simulink model "prova_ottimizzatore"  (R2018a)
settings: Solver=VariableStepAuto  StartTime=0.0  StopTime=10.0  RelTol=1e-3
settings Model: Creator=root  LastModifiedBy=root

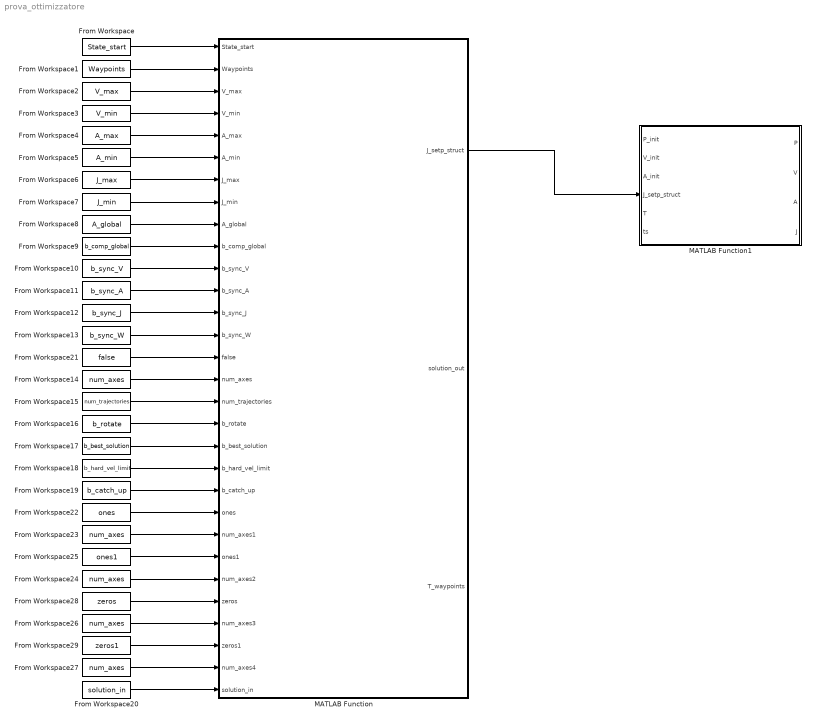
== system prova_ottimizzatore ==
  From Workspace : FromWorkspace  VariableName=State_start  SampleTime=0
  From Workspace1 : FromWorkspace  VariableName=Waypoints  SampleTime=0
  From Workspace10 : FromWorkspace  VariableName=b_sync_V  SampleTime=0
  From Workspace11 : FromWorkspace  VariableName=b_sync_A  SampleTime=0
  From Workspace12 : FromWorkspace  VariableName=b_sync_J  SampleTime=0
  From Workspace13 : FromWorkspace  VariableName=b_sync_W  SampleTime=0
  From Workspace{14,23..24,26..27} (5 alike) : FromWorkspace  VariableName=num_axes  SampleTime=0
  From Workspace15 : FromWorkspace  VariableName=num_trajectories  SampleTime=0
  From Workspace16 : FromWorkspace  VariableName=b_rotate  SampleTime=0
  From Workspace17 : FromWorkspace  VariableName=b_best_solution  SampleTime=0
  From Workspace18 : FromWorkspace  VariableName=b_hard_vel_limit  SampleTime=0
  From Workspace19 : FromWorkspace  VariableName=b_catch_up  SampleTime=0
  From Workspace2 : FromWorkspace  VariableName=V_max  SampleTime=0
  From Workspace20 : FromWorkspace  VariableName=solution_in  SampleTime=0
  From Workspace21 : FromWorkspace  VariableName=false  SampleTime=0
  From Workspace22 : FromWorkspace  VariableName=ones  SampleTime=0
  From Workspace25 : FromWorkspace  VariableName=ones1  SampleTime=0
  From Workspace28 : FromWorkspace  VariableName=zeros  SampleTime=0
  From Workspace29 : FromWorkspace  VariableName=zeros1  SampleTime=0
  From Workspace3 : FromWorkspace  VariableName=V_min  SampleTime=0
  From Workspace4 : FromWorkspace  VariableName=A_max  SampleTime=0
  From Workspace5 : FromWorkspace  VariableName=A_min  SampleTime=0
  From Workspace6 : FromWorkspace  VariableName=J_max  SampleTime=0
  From Workspace7 : FromWorkspace  VariableName=J_min  SampleTime=0
  From Workspace8 : FromWorkspace  VariableName=A_global  SampleTime=0
  From Workspace9 : FromWorkspace  VariableName=b_comp_global  SampleTime=0
  MATLAB Function : MATLAB Function  TreatAsAtomicUnit=on
  MATLAB Function1 : MATLAB Function  TreatAsAtomicUnit=on
  wires:
  From Workspace/1 -> MATLAB Function/1(State_start)
  From Workspace1/1 -> MATLAB Function/2(Waypoints)
  From Workspace2/1 -> MATLAB Function/3(V_max)
  From Workspace3/1 -> MATLAB Function/4(V_min)
  From Workspace4/1 -> MATLAB Function/5(A_max)
  From Workspace5/1 -> MATLAB Function/6(A_min)
  From Workspace6/1 -> MATLAB Function/7(J_max)
  From Workspace7/1 -> MATLAB Function/8(J_min)
  From Workspace8/1 -> MATLAB Function/9(A_global)
  From Workspace9/1 -> MATLAB Function/10(b_comp_global)
  From Workspace10/1 -> MATLAB Function/11(b_sync_V)
  From Workspace11/1 -> MATLAB Function/12(b_sync_A)
  From Workspace12/1 -> MATLAB Function/13(b_sync_J)
  From Workspace13/1 -> MATLAB Function/14(b_sync_W)
  From Workspace14/1 -> MATLAB Function/16(num_axes)
  From Workspace15/1 -> MATLAB Function/17(num_trajectories)
  From Workspace16/1 -> MATLAB Function/18(b_rotate)
  From Workspace17/1 -> MATLAB Function/19(b_best_solution)
  From Workspace18/1 -> MATLAB Function/20(b_hard_vel_limit)
  From Workspace19/1 -> MATLAB Function/21(b_catch_up)
  From Workspace20/1 -> MATLAB Function/30(solution_in)
  From Workspace21/1 -> MATLAB Function/15(false)
  From Workspace22/1 -> MATLAB Function/22(ones)
  From Workspace23/1 -> MATLAB Function/23(num_axes1)
  From Workspace24/1 -> MATLAB Function/25(num_axes2)
  From Workspace25/1 -> MATLAB Function/24(ones1)
  From Workspace26/1 -> MATLAB Function/27(num_axes3)
  From Workspace27/1 -> MATLAB Function/29(num_axes4)
  From Workspace28/1 -> MATLAB Function/26(zeros)
  From Workspace29/1 -> MATLAB Function/28(zeros1)
  MATLAB Function/1(J_setp_struct) -> MATLAB Function1/4(J_setp_struct)

== matlab function prova_ottimizzatore/MATLAB Function1 ==
  data: P_init input; P output; V_init input; A_init input; J_setp_struct input; T input; ts input; V output; A output; J output
function [P,V,A,J] = rollout(P_init,V_init,A_init,J_setp_struct,T,ts)

== matlab function prova_ottimizzatore/MATLAB Function ==
  data: State_start input; J_setp_struct output; Waypoints input; V_max input; V_min input; A_max input; A_min input; J_max input; J_min input; A_global input; b_comp_global input; b_sync_V input; b_sync_A input; b_sync_J input; b_sync_W input; false input; num_axes input; num_trajectories input; b_rotate input; b_best_solution input; b_hard_vel_limit input; b_catch_up input; ones input; num_axes1 input; ones1 input; num_axes2 input; zeros input; num_axes3 input; zeros1 input; num_axes4 input; solution_in input; solution_out output; T_waypoints output
function [J_setp_struct,solution_out,T_waypoints]=  opt_control_mex(State_start,Waypoints,V_max,V_min,A_max,A_min,J_max,J_min,A_global,b_comp_global,b_sync_V,b_sync_A,b_sync_J,b_sync_W,false,num_axes,num_trajectories,b_rotate, b_best_solution,b_hard_vel_limit,b_catch_up,ones,num_axes1,ones1,     num_axes2,zeros,   num_axes3,zeros1,   num_axes4,solution_in)
